simulink library "KALMAN_MASTER"  (Simulink 8.6)
settings: Solver=VariableStepAuto  StartTime=0.0  StopTime=10.0  RelTol=1e-3
libraries: cdsFilt x6, cdsMuxMatrix x4
settings Model: Creator=controls  LastModifiedBy=controls

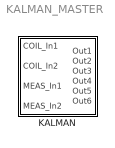
== system KALMAN_MASTER ==
  KALMAN : Subsystem

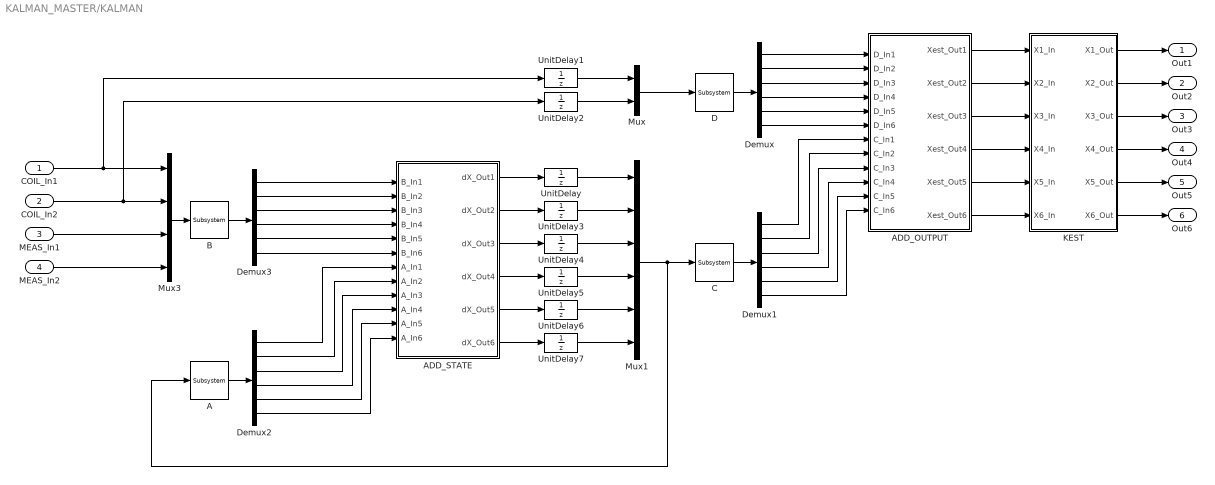
== system KALMAN_MASTER/KALMAN ==
  COIL_In1 : Inport
  COIL_In2 : Inport  Port=2
  MEAS_In1 : Inport  Port=3
  MEAS_In2 : Inport  Port=4
  A : cdsMuxMatrix/Subsystem  Tag=cdsMuxMatrix  Description=Any size matrix. Inputs and outputs must be connected using Mux and Demux parts.
      settings: AttributesFormatString=%<Tag>
  ADD_OUTPUT : Subsystem
  ADD_STATE : Subsystem
  B : cdsMuxMatrix/Subsystem  Tag=cdsMuxMatrix  Description=Any size matrix. Inputs and outputs must be connected using Mux and Demux parts.
      settings: AttributesFormatString=%<Tag>
  C : cdsMuxMatrix/Subsystem  Tag=cdsMuxMatrix  Description=Any size matrix. Inputs and outputs must be connected using Mux and Demux parts.
      settings: AttributesFormatString=%<Tag>
  D : cdsMuxMatrix/Subsystem  Tag=cdsMuxMatrix  Description=Any size matrix. Inputs and outputs must be connected using Mux and Demux parts.
      settings: AttributesFormatString=%<Tag>
  Demux{,1..3} (4 alike) : Demux  Outputs=6
  KEST : Subsystem
  Mux : Mux  Inputs=2
  Mux1 : Mux  Inputs=6
  Mux3 : Mux
  UnitDelay{,1..7} (8 alike) : UnitDelay
  Out1 : Outport
  Out2 : Outport  Port=2
  Out3 : Outport  Port=3
  Out4 : Outport  Port=4
  Out5 : Outport  Port=5
  Out6 : Outport  Port=6
  wires:
  D/1 -> Demux/1
  C/1 -> Demux1/1
  Mux/1 -> D/1
  Mux1/1 -> A/1, C/1
  A/1 -> Demux2/1
  Mux3/1 -> B/1
  B/1 -> Demux3/1
  UnitDelay2/1 -> Mux/2
  UnitDelay1/1 -> Mux/1
  UnitDelay5/1 -> Mux1/4
  UnitDelay4/1 -> Mux1/3
  UnitDelay3/1 -> Mux1/2
  UnitDelay6/1 -> Mux1/5
  UnitDelay7/1 -> Mux1/6
  UnitDelay/1 -> Mux1/1
  ADD_STATE/1(dX_Out1) -> UnitDelay/1
  ADD_STATE/2(dX_Out2) -> UnitDelay3/1
  ADD_STATE/3(dX_Out3) -> UnitDelay4/1
  ADD_STATE/4(dX_Out4) -> UnitDelay5/1
  ADD_STATE/5(dX_Out5) -> UnitDelay6/1
  ADD_STATE/6(dX_Out6) -> UnitDelay7/1
  COIL_In2/1 -> Mux3/2, UnitDelay2/1
  COIL_In1/1 -> Mux3/1, UnitDelay1/1
  Demux3/1 -> ADD_STATE/1(B_In1)
  Demux3/3 -> ADD_STATE/3(B_In3)
  Demux3/4 -> ADD_STATE/4(B_In4)
  Demux3/5 -> ADD_STATE/5(B_In5)
  Demux3/6 -> ADD_STATE/6(B_In6)
  Demux3/2 -> ADD_STATE/2(B_In2)
  Demux2/1 -> ADD_STATE/7(A_In1)
  Demux2/4 -> ADD_STATE/10(A_In4)
  Demux2/3 -> ADD_STATE/9(A_In3)
  Demux2/6 -> ADD_STATE/12(A_In6)
  Demux2/2 -> ADD_STATE/8(A_In2)
  Demux2/5 -> ADD_STATE/11(A_In5)
  Demux/1 -> ADD_OUTPUT/1(D_In1)
  Demux/5 -> ADD_OUTPUT/5(D_In5)
  Demux/4 -> ADD_OUTPUT/4(D_In4)
  Demux/2 -> ADD_OUTPUT/2(D_In2)
  Demux/3 -> ADD_OUTPUT/3(D_In3)
  Demux/6 -> ADD_OUTPUT/6(D_In6)
  Demux1/4 -> ADD_OUTPUT/10(C_In4)
  Demux1/5 -> ADD_OUTPUT/11(C_In5)
  Demux1/2 -> ADD_OUTPUT/8(C_In2)
  Demux1/3 -> ADD_OUTPUT/9(C_In3)
  Demux1/1 -> ADD_OUTPUT/7(C_In1)
  Demux1/6 -> ADD_OUTPUT/12(C_In6)
  MEAS_In1/1 -> Mux3/3
  MEAS_In2/1 -> Mux3/4
  ADD_OUTPUT/2(Xest_Out2) -> KEST/2(X2_In)
  ADD_OUTPUT/6(Xest_Out6) -> KEST/6(X6_In)
  ADD_OUTPUT/1(Xest_Out1) -> KEST/1(X1_In)
  ADD_OUTPUT/5(Xest_Out5) -> KEST/5(X5_In)
  ADD_OUTPUT/4(Xest_Out4) -> KEST/4(X4_In)
  ADD_OUTPUT/3(Xest_Out3) -> KEST/3(X3_In)
  KEST/5(X5_Out) -> Out5/1
  KEST/4(X4_Out) -> Out4/1
  KEST/2(X2_Out) -> Out2/1
  KEST/6(X6_Out) -> Out6/1
  KEST/1(X1_Out) -> Out1/1
  KEST/3(X3_Out) -> Out3/1

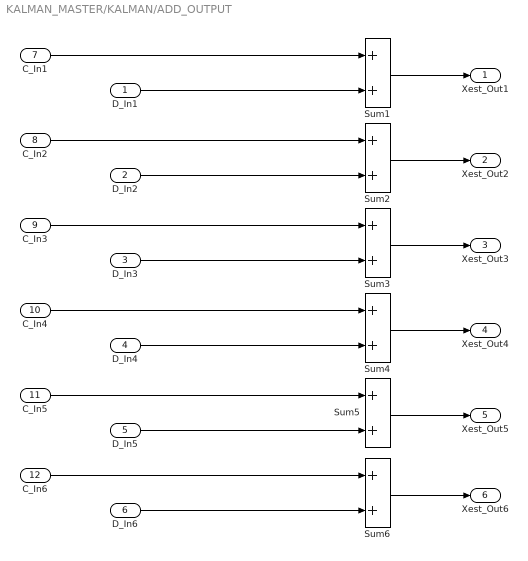
== system KALMAN_MASTER/KALMAN/ADD_OUTPUT ==
  D_In1 : Inport
  D_In2 : Inport  Port=2
  D_In3 : Inport  Port=3
  D_In4 : Inport  Port=4
  D_In5 : Inport  Port=5
  D_In6 : Inport  Port=6
  C_In1 : Inport  Port=7
  C_In2 : Inport  Port=8
  C_In3 : Inport  Port=9
  C_In4 : Inport  Port=10
  C_In5 : Inport  Port=11
  C_In6 : Inport  Port=12
  Sum{1..6} (6 alike) : Sum
  Xest_Out1 : Outport
  Xest_Out2 : Outport  Port=2
  Xest_Out3 : Outport  Port=3
  Xest_Out4 : Outport  Port=4
  Xest_Out5 : Outport  Port=5
  Xest_Out6 : Outport  Port=6
  wires:
  D_In2/1 -> Sum2/2
  D_In3/1 -> Sum3/2
  D_In4/1 -> Sum4/2
  D_In5/1 -> Sum5/2
  D_In6/1 -> Sum6/2
  D_In1/1 -> Sum1/2
  C_In5/1 -> Sum5/1
  C_In6/1 -> Sum6/1
  C_In4/1 -> Sum4/1
  C_In3/1 -> Sum3/1
  C_In2/1 -> Sum2/1
  C_In1/1 -> Sum1/1
  Sum6/1 -> Xest_Out6/1
  Sum5/1 -> Xest_Out5/1
  Sum4/1 -> Xest_Out4/1
  Sum3/1 -> Xest_Out3/1
  Sum2/1 -> Xest_Out2/1
  Sum1/1 -> Xest_Out1/1

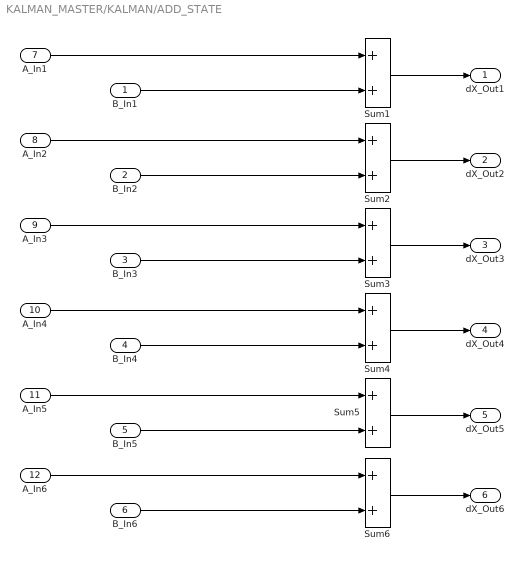
== system KALMAN_MASTER/KALMAN/ADD_STATE ==
  B_In1 : Inport
  B_In2 : Inport  Port=2
  B_In3 : Inport  Port=3
  B_In4 : Inport  Port=4
  B_In5 : Inport  Port=5
  B_In6 : Inport  Port=6
  A_In1 : Inport  Port=7
  A_In2 : Inport  Port=8
  A_In3 : Inport  Port=9
  A_In4 : Inport  Port=10
  A_In5 : Inport  Port=11
  A_In6 : Inport  Port=12
  Sum{1..6} (6 alike) : Sum
  dX_Out1 : Outport
  dX_Out2 : Outport  Port=2
  dX_Out3 : Outport  Port=3
  dX_Out4 : Outport  Port=4
  dX_Out5 : Outport  Port=5
  dX_Out6 : Outport  Port=6
  wires:
  Sum1/1 -> dX_Out1/1
  Sum2/1 -> dX_Out2/1
  Sum3/1 -> dX_Out3/1
  Sum4/1 -> dX_Out4/1
  Sum5/1 -> dX_Out5/1
  Sum6/1 -> dX_Out6/1
  A_In1/1 -> Sum1/1
  A_In2/1 -> Sum2/1
  A_In3/1 -> Sum3/1
  A_In4/1 -> Sum4/1
  A_In6/1 -> Sum6/1
  A_In5/1 -> Sum5/1
  B_In1/1 -> Sum1/2
  B_In6/1 -> Sum6/2
  B_In5/1 -> Sum5/2
  B_In4/1 -> Sum4/2
  B_In3/1 -> Sum3/2
  B_In2/1 -> Sum2/2

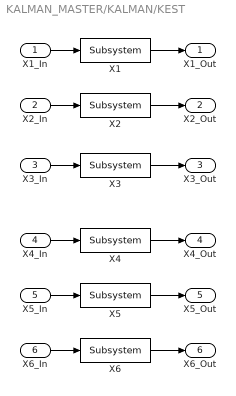
== system KALMAN_MASTER/KALMAN/KEST ==
  X1_In : Inport
  X2_In : Inport  Port=2
  X3_In : Inport  Port=3
  X4_In : Inport  Port=4
  X5_In : Inport  Port=5
  X6_In : Inport  Port=6
  X1 : cdsFilt/Subsystem  Tag=cdsFilt  Description=|
      | Purpose:                                                                                                                                                                                                                                  
      | Standard CDS IIR filter module.                                                                                                                                                                                                           
      |                                                                                                                                                                                                                                           
      | Operation:                                                                                                                                                                                                                                
      | Consists of 10 second order section IIR filters, plus a ramped gain stage. In FE code, also provides pre-defined test points and excitation channel inputs. The filter coefficients are defined in the LIGO system using the 'foton' tool.
      |                                                                                                                                                                                                                                           
      | Usage:                                                                                                                                                                                                                                    
      | Name the part with the desired filter module name.
      settings: AttributesFormatString=%<Tag>
  X2 : cdsFilt/Subsystem  Tag=cdsFilt  Description=|
      | Purpose:                                                                                                                                                                                                                                  
      | Standard CDS IIR filter module.                                                                                                                                                                                                           
      |                                                                                                                                                                                                                                           
      | Operation:                                                                                                                                                                                                                                
      | Consists of 10 second order section IIR filters, plus a ramped gain stage. In FE code, also provides pre-defined test points and excitation channel inputs. The filter coefficients are defined in the LIGO system using the 'foton' tool.
      |                                                                                                                                                                                                                                           
      | Usage:                                                                                                                                                                                                                                    
      | Name the part with the desired filter module name.
      settings: AttributesFormatString=%<Tag>
  X3 : cdsFilt/Subsystem  Tag=cdsFilt  Description=|
      | Purpose:                                                                                                                                                                                                                                  
      | Standard CDS IIR filter module.                                                                                                                                                                                                           
      |                                                                                                                                                                                                                                           
      | Operation:                                                                                                                                                                                                                                
      | Consists of 10 second order section IIR filters, plus a ramped gain stage. In FE code, also provides pre-defined test points and excitation channel inputs. The filter coefficients are defined in the LIGO system using the 'foton' tool.
      |                                                                                                                                                                                                                                           
      | Usage:                                                                                                                                                                                                                                    
      | Name the part with the desired filter module name.
      settings: AttributesFormatString=%<Tag>
  X4 : cdsFilt/Subsystem  Tag=cdsFilt  Description=|
      | Purpose:                                                                                                                                                                                                                                  
      | Standard CDS IIR filter module.                                                                                                                                                                                                           
      |                                                                                                                                                                                                                                           
      | Operation:                                                                                                                                                                                                                                
      | Consists of 10 second order section IIR filters, plus a ramped gain stage. In FE code, also provides pre-defined test points and excitation channel inputs. The filter coefficients are defined in the LIGO system using the 'foton' tool.
      |                                                                                                                                                                                                                                           
      | Usage:                                                                                                                                                                                                                                    
      | Name the part with the desired filter module name.
      settings: AttributesFormatString=%<Tag>
  X5 : cdsFilt/Subsystem  Tag=cdsFilt  Description=|
      | Purpose:                                                                                                                                                                                                                                  
      | Standard CDS IIR filter module.                                                                                                                                                                                                           
      |                                                                                                                                                                                                                                           
      | Operation:                                                                                                                                                                                                                                
      | Consists of 10 second order section IIR filters, plus a ramped gain stage. In FE code, also provides pre-defined test points and excitation channel inputs. The filter coefficients are defined in the LIGO system using the 'foton' tool.
      |                                                                                                                                                                                                                                           
      | Usage:                                                                                                                                                                                                                                    
      | Name the part with the desired filter module name.
      settings: AttributesFormatString=%<Tag>
  X6 : cdsFilt/Subsystem  Tag=cdsFilt  Description=|
      | Purpose:                                                                                                                                                                                                                                  
      | Standard CDS IIR filter module.                                                                                                                                                                                                           
      |                                                                                                                                                                                                                                           
      | Operation:                                                                                                                                                                                                                                
      | Consists of 10 second order section IIR filters, plus a ramped gain stage. In FE code, also provides pre-defined test points and excitation channel inputs. The filter coefficients are defined in the LIGO system using the 'foton' tool.
      |                                                                                                                                                                                                                                           
      | Usage:                                                                                                                                                                                                                                    
      | Name the part with the desired filter module name.
      settings: AttributesFormatString=%<Tag>
  X1_Out : Outport
  X2_Out : Outport  Port=2
  X3_Out : Outport  Port=3
  X4_Out : Outport  Port=4
  X5_Out : Outport  Port=5
  X6_Out : Outport  Port=6
  wires:
  X3/1 -> X3_Out/1
  X4/1 -> X4_Out/1
  X5/1 -> X5_Out/1
  X3_In/1 -> X3/1
  X4_In/1 -> X4/1
  X5_In/1 -> X5/1
  X6/1 -> X6_Out/1
  X1/1 -> X1_Out/1
  X2/1 -> X2_Out/1
  X6_In/1 -> X6/1
  X1_In/1 -> X1/1
  X2_In/1 -> X2/1
